simulink model "LQR_demo"  (R2020b)
settings: Solver=ode4  StartTime=0.0  StopTime=10  FixedStep=0.01  RelTol=1e-3
settings Model: Creator=xzh123  LastModifiedBy=xzh123

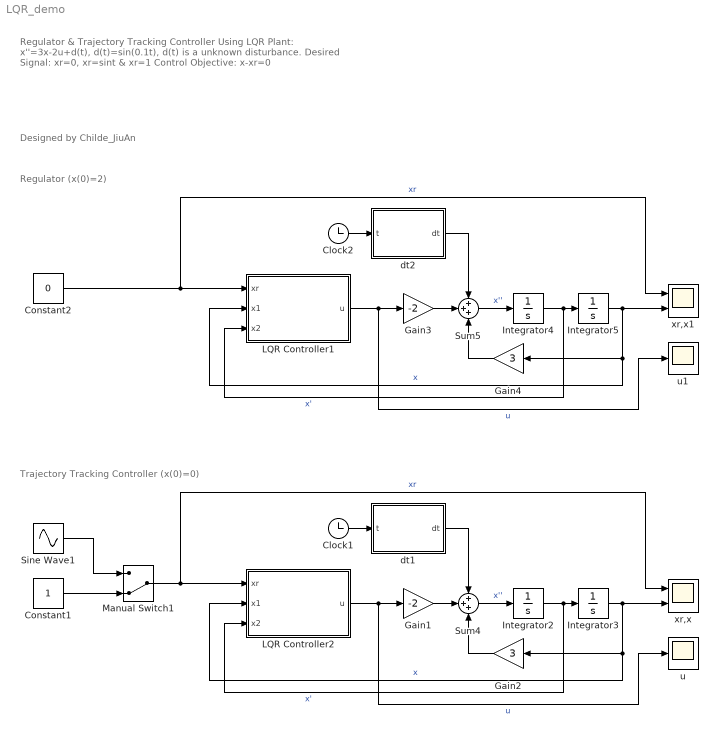
== system LQR_demo ==
  note: Trajectory Tracking Controller (x(0)=0)
  note: Designed by Childe_JiuAn
  note: Regulator & Trajectory Tracking Controller Using LQR
      |
      | Plant: x''=3x-2u+d(t), d(t)=sin(0.1t), d(t) is a unknown disturbance.
      |
      | Desired Signal: xr=0, xr=sint & xr=1
      |
      | Control Objective: x-xr=0
  note: Regulator (x(0)=2)
  Clock1 : Clock
  Clock2 : Clock
  Constant1 : Constant
  Constant2 : Constant  Value=0
  Gain1 : Gain  Gain=-2
  Gain2 : Gain  Gain=3
  Gain3 : Gain  Gain=-2
  Gain4 : Gain  Gain=3
  Integrator2 : Integrator
  Integrator3 : Integrator
  Integrator4 : Integrator
  Integrator5 : Integrator  InitialCondition=2
  LQR Controller1 : MATLAB Function  TreatAsAtomicUnit=on
  LQR Controller2 : MATLAB Function  TreatAsAtomicUnit=on
  Manual Switch1 : ManualSwitch  CurrentSetting=0
  Sine Wave1 : Sin  Frequency=3  SampleTime=0
  Sum4 : Sum  Inputs=+++
  Sum5 : Sum  Inputs=+++
  dt1 : MATLAB Function  TreatAsAtomicUnit=on
  dt2 : MATLAB Function  TreatAsAtomicUnit=on
  u : Scope
  u1 : Scope
  xr,x : Scope  NumInputPorts=2
  xr,x1 : Scope  NumInputPorts=2
  wires:
  Constant1/1 -> Manual Switch1/2
  Sine Wave1/1 -> Manual Switch1/1
  LQR Controller2/1(u) -> u/1, Gain1/1  "u"
  Integrator3/1 -> LQR Controller2/2(x1), Gain2/1, xr,x/2  "x"
  Sum4/1 -> Integrator2/1  "x''"
  Gain1/1 -> Sum4/2
  Integrator2/1 -> LQR Controller2/3(x2), Integrator3/1  "x'"
  Clock1/1 -> dt1/1(t)
  Gain2/1 -> Sum4/3
  Manual Switch1/1 -> xr,x/1, LQR Controller2/1(xr)  "xr"
  dt1/1(dt) -> Sum4/1
  dt2/1(dt) -> Sum5/1
  Constant2/1 -> xr,x1/1, LQR Controller1/1(xr)  "xr"
  Gain3/1 -> Sum5/2
  Sum5/1 -> Integrator4/1  "x''"
  Gain4/1 -> Sum5/3
  Clock2/1 -> dt2/1(t)
  LQR Controller1/1(u) -> u1/1, Gain3/1  "u"
  Integrator4/1 -> LQR Controller1/3(x2), Integrator5/1  "x'"
  Integrator5/1 -> LQR Controller1/2(x1), Gain4/1, xr,x1/2  "x"

== matlab function LQR_demo/LQR Controller1 ==
  data: xr input; u output; x1 input; x2 input
function u = LQR(xr,x1,x2)

% state space
 A = [0 1;
      3 0];
 B = [0;
     -2];

 % weight matrix
 Q = [100 0
      0   1];
 R = 0.01;
 
 % control law
 coder.extrinsic('lqr');
 K = zeros(1,2);
 K = lqr(A,B,Q,R);
 u = 0;
 u = -K(1)*x1-K(2)*x2;
end

== matlab function LQR_demo/dt1 ==
  data: t input; dt output
function dt = fcn(t)

d=sin(0.1*t);

== matlab function LQR_demo/dt2 ==
  data: t input; dt output
function dt = fcn(t)

d=sin(0.1*t);

== matlab function LQR_demo/LQR Controller2 ==
  data: xr input; u output; x1 input; x2 input
function u = LQR(xr,x1,x2)

% state space
 A = [0 1;
      3 0];
 B = [0;
     -2];

 % weight matrix
 Q = [100 0
      0   1];
 R = 0.01;
 
 % control law
 coder.extrinsic('lqr');
 K = zeros(1,2);
 K = lqr(A,B,Q,R);
 u = 0;
 u = -K(1)*x1-K(2)*x2+(3/2+K(1))*xr;
end
